simulink model "buoi1"  (R2020b)
settings: Solver=VariableStepAuto  StartTime=0.0  StopTime=10.0  RelTol=1e-3
libraries: dsparch4 x1
settings Model: Creator=htn  LastModifiedBy=htn

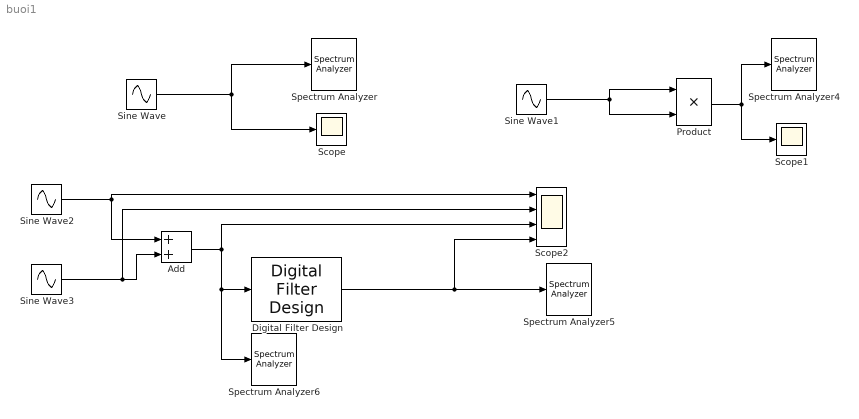
== system buoi1 ==
  Add : Sum
  Digital Filter Design : dsparch4/Digital Filter Design  mwdsp_browser_bugfix_var=off
  Product : Product
  Scope : Scope
  Scope1 : Scope
  Scope2 : Scope  NumInputPorts=4
  Sine Wave : Sin  Frequency=2*pi*1000  SampleTime=1/100000
  Sine Wave1 : Sin  Frequency=2*pi*1000  SampleTime=1/100000
  Sine Wave2 : Sin  Frequency=2*pi*1000  SampleTime=1/50000
  Sine Wave3 : Sin  Frequency=2*pi*3000  SampleTime=1/50000
  Spectrum Analyzer{,4..6} (4 alike) : SpectrumAnalyzer
  wires:
  Sine Wave/1 -> Spectrum Analyzer/1, Scope/1
  Product/1 -> Scope1/1, Spectrum Analyzer4/1
  Sine Wave1/1 -> Product/1, Product/2
  Sine Wave2/1 -> Add/1, Scope2/1
  Sine Wave3/1 -> Scope2/2, Add/2
  Add/1 -> Scope2/3, Spectrum Analyzer6/1, Digital Filter Design/1
  Digital Filter Design/1 -> Scope2/4, Spectrum Analyzer5/1
